simulink model "c28035solar_inverter"  (R2021b)
settings: Solver=FixedStepDiscrete  StartTime=0.0  StopTime=inf  FixedStep=1e-5  RelTol=1e-3  EnableMultiTasking=on
undefined symbols (not defined in the file or in its folder): Down, GPTRIP1SEL, GPTRIP2SEL, TZ1, TZ2, Up
libraries: c2802xlib x8, tiiqmathlib x6, simulink x5, c280xlib x3, c28xdmclib x2, c2000lib x1, demo_controls x1
settings Model: ExtModeTrigType=signal  ExtModeTrigDuration=10  ExtModeTrigDurationFloating=10  ExtModeTrigDelay=-2  ExtModeTrigDirection=either  ExtModeTrigLevel=0.500000  Creator=The MathWorks, Inc.  LastModifiedBy=The MathWorks, Inc.
settings SolverCC: AlgebraicLoopSolver=TrustRegion
settings DataIOCC: LimitDataPoints=on  SaveFormat=Array  SaveOutput=off  SaveTime=off  ReturnWorkspaceOutputs=off
settings OptimizationCC: DefaultParameterBehavior=Inlined  UseSpecifiedMinMax=on  StrengthReduction=on  PassReuseOutputArgsAs=Individual arguments  NoFixptDivByZeroProtection=on  EfficientFloat2IntCast=on  LifeSpan=1  MaxStackSize=512  EfficientTunableParamExpr=on
settings DebuggingCC: SolverPrmCheckMsg=warning  InheritedTsInSrcMsg=none  ParameterPrecisionLossMsg=none  AllowSymbolicDim=off  SFUnexpectedBacktrackingDiag=warning  SFNoUnconditionalDefaultTransitionDiag=warning  SFExecutionAtInitializationDiag=none  SFMachineParentedDataDiag=warning  ArithmeticOperatorsInVariantConditions=warning
settings HardwareCC: ProdBitPerChar=16  ProdBitPerInt=16  ProdBitPerPointer=16  ProdBitPerSizeT=32  ProdBitPerPtrDiffT=32  ProdLargestAtomicInteger=Integer  ProdLargestAtomicFloat=None  ProdWordSize=16  ProdHWDeviceType=Texas Instruments->C2000
settings ModelReferenceCC: PropagateSignalLabelsOutOfModel=off
settings SFSimCC: SimUseLocalCustomCode=off  MATLABDynamicMemAlloc=off  CustomCodeUndefinedFunction=UseInterfaceOnly
settings RTWCC: Description=Embedded Coder  SystemTargetFile=ert.tlc  HardwareBoard=TI Piccolo F2803x  TemplateMakefile=ert_default_tmf  RTWUseLocalCustomCode=off  Toolchain=Texas Instruments Code Composer Studio (C2000)  BuildConfiguration=Debug
settings CodeAppCC: IgnoreCustomStorageClasses=off  StateflowObjectComments=on
settings ERTTargetCC: CodeReplacementLibrary=TI C28x  UtilityFuncGeneration=Shared location  MultiwordLength=2048  CombineSignalStateStructs=on  SupportNonFinite=off  SupportComplex=off  SupportContinuousTime=on  ExtModeMexFile=TIC2000ExternalModeOpen  ExtModeMexArgs=1 65 115385 30  ExtModeIntrfLevel=Level2 - Open  ERTFilePackagingFormat=Compact  MemSecPackage=tic2000demospkg  MemSecFuncExecute=code_ramfuncs
settings ConfigComp: CovMetricSettings=dw  CovSaveCumulativeToWorkspaceVar=on  CovSaveSingleToWorkspaceVar=on  CovExternalEMLEnable=off  CovSFcnEnable=off
settings SimscapeCC: SimscapeNormalizeSystem=off
settings ConfigurationSet: Description=SimMechanics 2G

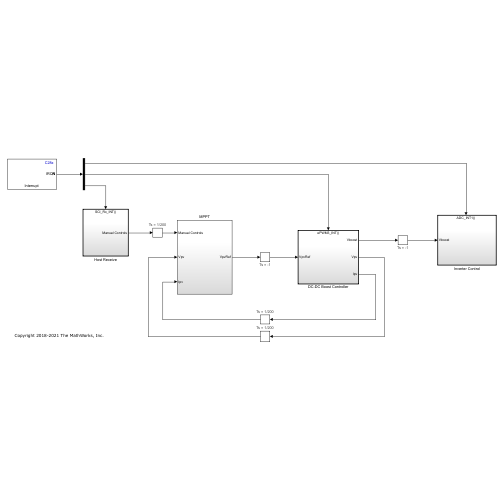
[thumbnail: Simulink's stored preview of the top-level diagram]
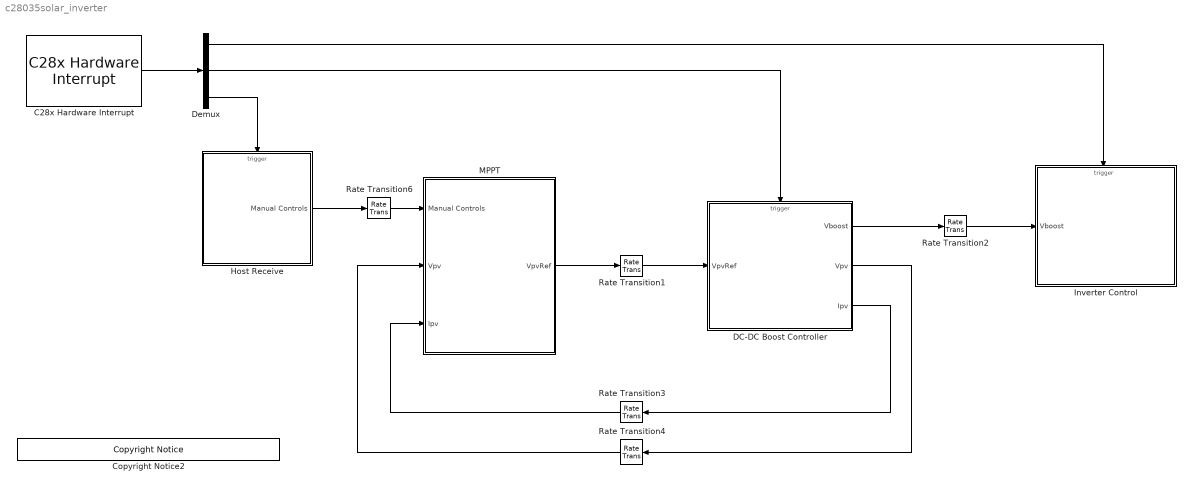
== system c28035solar_inverter ==
  C28x Hardware Interrupt : c2000lib/Scheduling/C28x Hardware Interrupt  irqnumbers=[1 3 9]  pienumbers=[1 3 1]  irqpriorities=[36 30 50]  irqpreempts=[1 0 0]  showinput=off  dspchiptype=C280X
      settings: SourceProductBaseCode=TIC2000
  Copyright Notice2 : demo_controls/Copyright Notice  year=2018  prod=tic2000
      settings: SourceProductBaseCode=ME
  DC-DC Boost Controller : Subsystem  TreatAsAtomicUnit=on
  Demux : Demux  Outputs=3
  Host Receive : Subsystem
  Inverter Control : Subsystem  TreatAsAtomicUnit=on
  MPPT : Subsystem
  Rate Transition1 : RateTransition  Deterministic=off
      settings: AttributesFormatString=Ts = %<OutPortSampleTime>
  Rate Transition2 : RateTransition  Deterministic=off
      settings: AttributesFormatString=Ts = %<OutPortSampleTime>
  Rate Transition3 : RateTransition  Deterministic=off  OutPortSampleTime=1/200
      settings: AttributesFormatString=Ts = %<OutPortSampleTime>
  Rate Transition4 : RateTransition  Deterministic=off  OutPortSampleTime=1/200
      settings: AttributesFormatString=Ts = %<OutPortSampleTime>
  Rate Transition6 : RateTransition  Deterministic=off  OutPortSampleTime=1/200
      settings: AttributesFormatString=Ts = %<OutPortSampleTime>
  wires:
  DC-DC Boost Controller/1(Vboost) -> Rate Transition2/1
  Demux/2 -> DC-DC Boost Controller/Trigger
  Rate Transition2/1 -> Inverter Control/1(Vboost)
  Demux/3 -> Host Receive/Trigger
  Rate Transition3/1 -> MPPT/3(Ipv)
  Rate Transition4/1 -> MPPT/2(Vpv)
  C28x Hardware Interrupt/1 -> Demux/1
  Host Receive/1(Manual Controls) -> Rate Transition6/1
  DC-DC Boost Controller/3(Ipv) -> Rate Transition3/1
  DC-DC Boost Controller/2(Vpv) -> Rate Transition4/1
  Rate Transition6/1 -> MPPT/1(Manual Controls)
  MPPT/1(VpvRef) -> Rate Transition1/1
  Demux/1 -> Inverter Control/Trigger
  Rate Transition1/1 -> DC-DC Boost Controller/1(VpvRef)

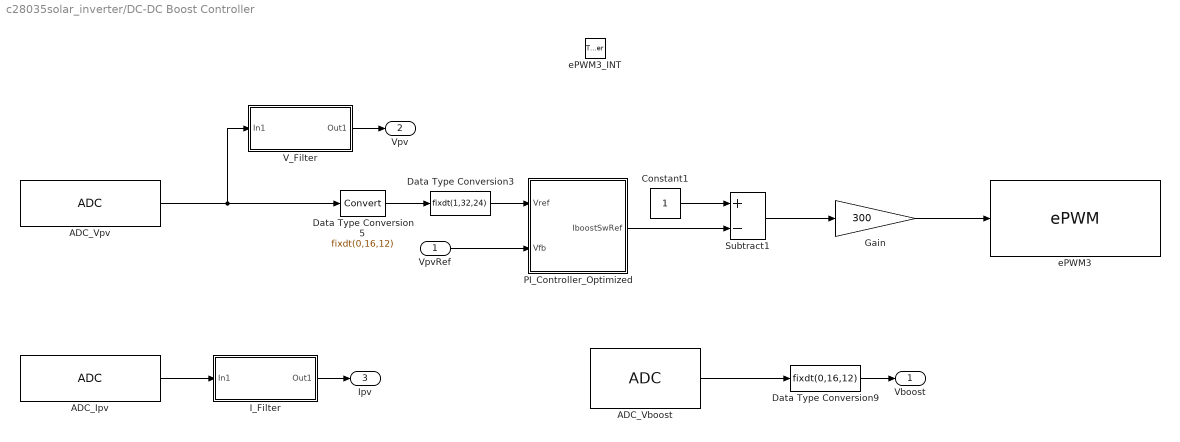
== system c28035solar_inverter/DC-DC Boost Controller ==
  VpvRef : Inport
  ePWM3_INT : TriggerPort  TriggerType=function-call  VariantControl=(inherit)
  ADC_Ipv : c2802xlib/ADC  blkParamProc=C2000  ADCModule=1  samplingMode=Single sample mode  ADCResolution=12-bit (Single-ended input)  useSOC1=SOC6  useSOC2=SOC0_SOC1  SOCAcquisitionWindow=7  SOCTriggerSource=ePWM3_ADCSOCA  SOCInterruptTrigger=No ADCINT  Ts=-1  dType=uint16  postInterrupt=off  interruptSel=ADCINT1  ADCINTContinuous=off  endma=off  chdma=1  conv1=ADCINA0  conv2=ADCINA0 and ADCINB0  conv1_Type4=ADCIN0  conv2_Type4=ADCIN0 and ADCIN1
  ADC_Vboost : c2802xlib/ADC  blkParamProc=C2000  ADCModule=1  samplingMode=Single sample mode  ADCResolution=12-bit (Single-ended input)  useSOC1=SOC5  useSOC2=SOC0_SOC1  SOCAcquisitionWindow=7  SOCTriggerSource=ePWM3_ADCSOCB  SOCInterruptTrigger=No ADCINT  Ts=-1  dType=uint16  postInterrupt=off  interruptSel=ADCINT1  ADCINTContinuous=off  endma=off  chdma=1  conv1=ADCINA2  conv2=ADCINA0 and ADCINB0  conv1_Type4=ADCIN0  conv2_Type4=ADCIN0 and ADCIN1
  ADC_Vpv : c2802xlib/ADC  blkParamProc=C2000  ADCModule=1  samplingMode=Single sample mode  ADCResolution=12-bit (Single-ended input)  useSOC1=SOC7  useSOC2=SOC0_SOC1  SOCAcquisitionWindow=7  SOCTriggerSource=ePWM3_ADCSOCA  SOCInterruptTrigger=No ADCINT  Ts=-1  dType=uint16  postInterrupt=off  interruptSel=ADCINT1  ADCINTContinuous=on  endma=off  chdma=1  conv1=ADCINA1  conv2=ADCINA0 and ADCINB0  conv1_Type4=ADCIN0  conv2_Type4=ADCIN0 and ADCIN1
  Constant1 : Constant  OutDataTypeStr=fixdt(1,32,24)  SampleTime=-1
  Data Type Conversion3 : DataTypeConversion  OutDataTypeStr=fixdt(1,32,24)
  Data Type Conversion5 : DataTypeConversion  OutDataTypeStr=fixdt(0,16,12)  ConvertRealWorld=Stored Integer (SI)  RndMeth=Simplest
      settings: AttributesFormatString=DataType = %<OutDataTypeStr>
  Data Type Conversion9 : DataTypeConversion  OutDataTypeStr=fixdt(0,16,12)  ConvertRealWorld=Stored Integer (SI)  RndMeth=Simplest
      settings: AttributesFormatString=DataType = %<OutDataTypeStr>
  Gain : Gain  Gain=300  ParamDataTypeStr=uint16  OutDataTypeStr=uint16  RndMeth=Simplest
  I_Filter : Subsystem
  PI_Controller_Optimized : Subsystem  VariantControl=Variant
  Subtract1 : Sum  Inputs=+-
  V_Filter : Subsystem
  ePWM3 : c2802xlib/ePWM  PwmType=C2000  useModule=ePWM3  ePWMxLINKTBPRD=Not Linked  periodUnits=Clock cycles  timerSource=Specify via dialog  timerPeriod_clk=300  timerPeriod_sec=0.0001  tbshadow=Counter equals to zero  countingMode=Up-Down  phaseActiveEnable=Set counter to phase value specified via dialog  phaseDirection=Count up after sync  phaseActive=4  synchronizationEnable=off  dcaevt1Sync=off  dcbevt1Sync=off  synchronizationOption=Disable  perSynchronizationOption=Counter equals to period (CTR=PRD)  clockPrescale=1  HSclockPrescale=1  enswap=off  ePWMxAStatus=on  ePWMxAactionLogic1=Do nothing  ePWMxAactionLogic2=Do nothing  ePWMxAactionLogic3=Set  ePWMxAactionLogic4=Clear  ePWMxAactionLogic5=Do nothing  ePWMxAactionLogic6=Do nothing  ePWMxACSFenable=off  ePWMxACSFvalue=Forcing disable  ePWMxASFreload=Zero  ePWMxBStatus=off  ePWMxBactionLogic1=Do nothing  ePWMxBactionLogic2=Do nothing  ePWMxBactionLogic3=Do nothing  ePWMxBactionLogic4=Do nothing  ePWMxBactionLogic5=Do nothing  ePWMxBactionLogic6=Do nothing  ePWMxBCSFenable=off  ePWMxBCSFvalue=Forcing disable  ePWMxBSFreload=Zero  ePWNxBOutWay=off  ePWMxLINKCMPA=Not Linked  CMPAUnits=Clock cycles  CMPASource=Input port  CMPAValue_per=0  CMPAValue_clk=300  enCMPAshadow=Counter equals to zero (CTR=Zero)  ePWMxLINKCMPB=Not Linked  CMPBUnits=Clock cycles  CMPBSource=Specify via dialog  CMPBValue_per=50  CMPBValue_clk=0  enCMPBshadow=Counter equals to zero (CTR=Zero)  ePWMxLINKCMPC=Not Linked  CMPCUnits=Clock cycles  CMPCSource=Specify via dialog  CMPCValue_per=50  CMPCValue_clk=32000  enCMPCshadow=Counter equals to zero (CTR=Zero)  ePWMxLINKCMPD=Not Linked  CMPDUnits=Clock cycles  CMPDSource=Specify via dialog  CMPDValue_per=50  CMPDValue_clk=32000  enCMPDshadow=Counter equals to zero (CTR=Zero)  enableDBePWMxA=on  enableDBePWMxB=on  enhalfcycle=off  DBpolarity=Active high (AH)  DBedgeDelay=Positive  DBSource_ePWMxA=ePWMxA  DBSource_ePWMxB=ePWMxA  DBPeriodUnits=Clock cycles  DBperiodSource=Specify via dialog  REDperiod=0  FEDperiod=30  REDperiod_sec=0  FEDperiod_sec=0  LoadModeDBRED=Immediate without using shadow  LoadModeDBFED=Immediate without using shadow  adcstartModuleA=on  adcrequestEventA=Second event  adcstartEventA=Counter is incrementing and equals to the compare B register (CTRU=CMPB)  adcstartEventA_type2=Digital Compare Module A Event 1 start of conversion (DCAEVT1.soc)  adcstartModuleB=on  adcrequestEventB=Second event  adcstartEventB=Counter equals to period (CTR=PRD)  adcstartEventB_type2=Counter equals to zero (CTR=Zero)  intEn=on  intPrd=Second event  intSel=Counter equals to period (CTR=PRD)  intSel_type2=Counter equals to zero (CTR=Zero)  hrpe=off  enHRPWM=off  HRPWM_LoadMode=Counter equals to period (CTR=PRD)  HRPWM_CTLMode=Duty or Period control mode  HRPWM_EDGMode=Falling edge  hrpeb=off  enHRPWMB=off  HRPWM_LoadModeB=Counter equals to zero (CTR=ZERO)  HRPWM_CTLModeB=Duty or Period control mode  HRPWM_EDGModeB=Both edge  enHRDBRED=off  enHRDBFED=off  enSFO=off  enautoconv=off  chopperEnable=off  chopperFrequency=1  chopperFirstwidth=1  chopperDuty=12.5%  tripZonesource=Specify via dialog  tzselOSHT1=off  tzselOSHT2=off  tzselOSHT3=off  tzselOSHDCAEV1=off  tzselOSHDCBEV1=off  tzselCBC1=off  tzselCBC2=off  tzselCBC3=off  tzselCBCDCAEV2=off  tzselCBCDCBEV2=off  tzselOSHT4=off  tzselOSHT5=off  tzselOSHT6=off  tzselCBC4=off  tzselCBC5=off  tzselCBC6=off  enTzOstIntr=off  enTzCbcIntr=off  enTzDCAEVT1Intr=off  enTzDCAEVT2Intr=off  enTzDCBEVT1Intr=off  enTzDCBEVT2Intr=off  ePWMxAforced=Low  ePWMxBforced=No action  DCAEVT1forced=No action  DCBEVT1forced=No action  DCAEVT2forced=No action  DCBEVT2forced=No action  dcah=COMP1OUT input  dcal=COMP1OUT input  dcbh=COMP2OUT input  dcbl=COMP3OUT input  dcah_type2=GPTRIP1SEL/(TZ1)  dcal_type2=GPTRIP2SEL/(TZ2)  dcbh_type2=GPTRIP1SEL/(TZ1)  dcbl_type2=GPTRIP2SEL/(TZ2)  gendcaevt1=DCAH=high and DCAL=don't care  gendcaevt2=Event disabled  gendcbevt1=Event disabled  gendcbevt2=Event disabled  dcaevt1src=DCAEVT1 with async  dcaevt2src=DCAEVT2 with sync  dcbevt1src=DCBEVT1 with sync  dcbevt2src=DCBEVT2 with sync  pulsesel=Counter equals to zero (CTR=Zero)  blankinv=off  blankoffset=0  blankwidth=0  evsrcsel=Filtered version of DCAEVT1 (DCAEVT1FILT)  encape=off
  Vboost : Outport  VectorParamsAs1DForOutWhenUnconnected=off
  Vpv : Outport  Port=2  VectorParamsAs1DForOutWhenUnconnected=off
  Ipv : Outport  Port=3  VectorParamsAs1DForOutWhenUnconnected=off
  wires:
  Gain/1 -> ePWM3/1
  ADC_Vboost/1 -> Data Type Conversion9/1
  Data Type Conversion5/1 -> Data Type Conversion3/1
  Data Type Conversion3/1 -> PI_Controller_Optimized/1(Vref)
  ADC_Ipv/1 -> I_Filter/1(In1)
  ADC_Vpv/1 -> V_Filter/1(In1), Data Type Conversion5/1
  I_Filter/1(Out1) -> Ipv/1
  Data Type Conversion9/1 -> Vboost/1
  VpvRef/1 -> PI_Controller_Optimized/2(Vfb)
  V_Filter/1(Out1) -> Vpv/1
  Constant1/1 -> Subtract1/1
  PI_Controller_Optimized/1(IboostSwRef) -> Subtract1/2
  Subtract1/1 -> Gain/1

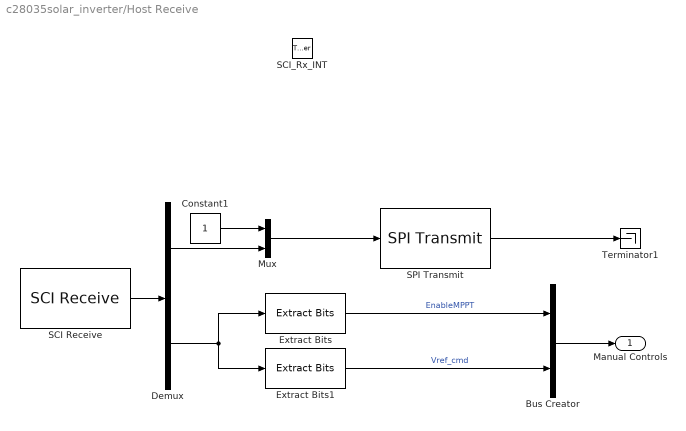
== system c28035solar_inverter/Host Receive ==
  SCI_Rx_INT : TriggerPort  TriggerType=function-call  VariantControl=Variant  PortDimensions=1
  Bus Creator : BusCreator  Inputs=2
  Constant1 : Constant  OutDataTypeStr=uint16  SampleTime=-1
  Demux : Demux  Outputs=2
  Extract Bits : simulink/Logic and Bit Operations/Extract Bits  bitsToExtract=Upper half  numBits=8  bitIdxRange=[0 7]  outScalingMode=Treat bit field as an integer
  Extract Bits1 : simulink/Logic and Bit Operations/Extract Bits  bitsToExtract=Lower half  numBits=8  bitIdxRange=[0 7]  outScalingMode=Treat bit field as an integer
  Mux : Mux  Inputs=2
  SCI Receive : c280xlib/SCI Receive  sciModule=A  dataHead=''  dataTail=''  dataType=uint16  dataDim=2  initValue=0  errOption=Output the last received value  errValue=0  sampleTime=-1  outputStatus=off  postInterrupt=on  numFifo=4
      settings: SourceProductBaseCode=TIC2000
  SPI Transmit : c280xlib/SPI Transmit  SPISelect=SPI_B  ClockPolarity=Rising_edge  ClockPhase=No_delay  SPIModule=uint32(0)  Mode=Master  BusSpeed=uint32(1000000)  FirstBitToTransfer=Most significant bit (MSB)  ClockMode=0  BlockFunction=Write  EnableRegisterAddress=on  RegisterAddress=0  OutputDataType=int8  OutputDataLength=1  BlockingMode=off  DataBits=16  UseCustomSSPin=Provided by the SPI peripheral  ActiveLowSSPin=Active low  Pin=0
      settings: SourceProductBaseCode=TIC2000
  Terminator1 : Terminator
  Manual Controls : Outport  VectorParamsAs1DForOutWhenUnconnected=off
  wires:
  Constant1/1 -> Mux/1
  Mux/1 -> SPI Transmit/1
  SPI Transmit/1 -> Terminator1/1
  Demux/2 -> Extract Bits/1, Extract Bits1/1
  Extract Bits/1 -> Bus Creator/1  "EnableMPPT"
  Extract Bits1/1 -> Bus Creator/2  "Vref_cmd"
  Bus Creator/1 -> Manual Controls/1
  SCI Receive/1 -> Demux/1
  Demux/1 -> Mux/2

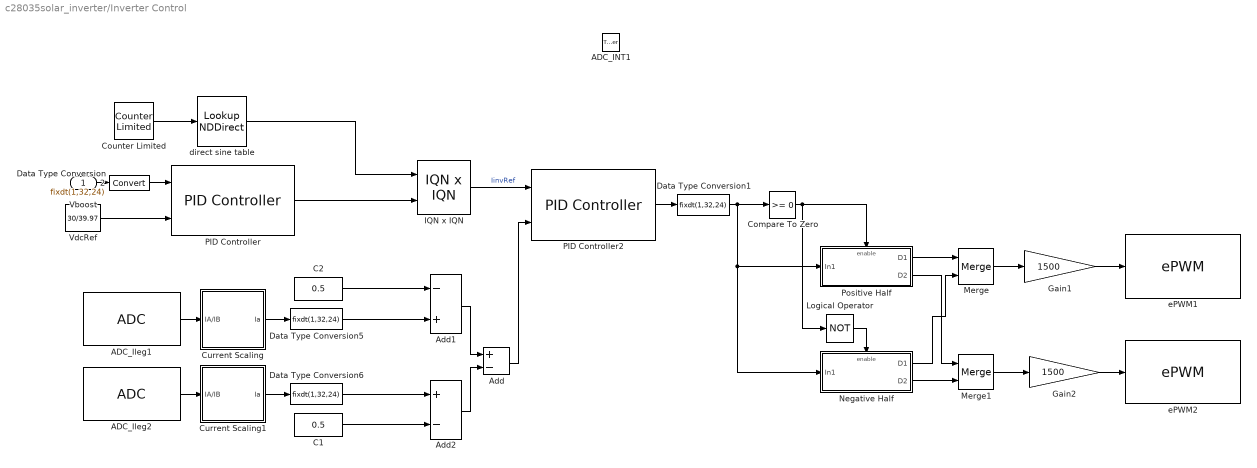
== system c28035solar_inverter/Inverter Control ==
  Vboost : Inport
  ADC_INT1 : TriggerPort  TriggerType=function-call  VariantControl=(inherit)
  ADC_Ileg1 : c2802xlib/ADC  blkParamProc=C2000  ADCModule=1  samplingMode=Single sample mode  ADCResolution=12-bit (Single-ended input)  useSOC1=SOC3  useSOC2=SOC0_SOC1  SOCAcquisitionWindow=7  SOCTriggerSource=ePWM1_ADCSOCA  SOCInterruptTrigger=No ADCINT  Ts=-1  dType=uint16  postInterrupt=on  interruptSel=ADCINT1  ADCINTContinuous=on  endma=off  chdma=1  conv1=ADCINA4  conv2=ADCINA0 and ADCINB0  conv1_Type4=ADCIN0  conv2_Type4=ADCIN0 and ADCIN1
  ADC_Ileg2 : c2802xlib/ADC  blkParamProc=C2000  ADCModule=1  samplingMode=Single sample mode  ADCResolution=12-bit (Single-ended input)  useSOC1=SOC4  useSOC2=SOC0_SOC1  SOCAcquisitionWindow=7  SOCTriggerSource=ePWM1_ADCSOCA  SOCInterruptTrigger=No ADCINT  Ts=-1  dType=uint16  postInterrupt=off  interruptSel=ADCINT1  ADCINTContinuous=off  endma=off  chdma=1  conv1=ADCINA6  conv2=ADCINA0 and ADCINB0  conv1_Type4=ADCIN0  conv2_Type4=ADCIN0 and ADCIN1
  Add : Sum  Inputs=+-
  Add1 : Sum  Inputs=-+
  Add2 : Sum  Inputs=+-
  C1 : Constant  Value=0.5  OutDataTypeStr=fixdt(1,32,24)  SampleTime=-1
  C2 : Constant  Value=0.5  OutDataTypeStr=fixdt(1,32,24)  SampleTime=-1
  Compare To Zero : simulink/Logic and Bit Operations/Compare To Zero  relop=>=  OutDataTypeStr=boolean
  Counter Limited : simulink/Sources/Counter Limited  uplimit=400  tsamp=-1
  Current Scaling : Subsystem
  Current Scaling1 : Subsystem
  Data Type Conversion1 : DataTypeConversion  OutDataTypeStr=fixdt(1,32,24)
  Data Type Conversion2 : DataTypeConversion  OutDataTypeStr=fixdt(1,32,24)
  Data Type Conversion5 : DataTypeConversion  OutDataTypeStr=fixdt(1,32,24)  ConvertRealWorld=Stored Integer (SI)
  Data Type Conversion6 : DataTypeConversion  OutDataTypeStr=fixdt(1,32,24)  ConvertRealWorld=Stored Integer (SI)
  Gain1 : Gain  Gain=1500  ParamDataTypeStr=uint16  OutDataTypeStr=uint16  RndMeth=Simplest
  Gain2 : Gain  Gain=1500  ParamDataTypeStr=uint16  OutDataTypeStr=uint16  RndMeth=Simplest
  IQN x IQN : tiiqmathlib/IQN x IQN  multiplyOption=Multiply
      settings: SourceProductBaseCode=TIC2000
  Logical Operator : Logic  Operator=NOT  AllPortsSameDT=off  OutDataTypeStr=boolean
  Merge : Merge
  Merge1 : Merge
  Negative Half : Subsystem  TreatAsAtomicUnit=on
  PID Controller : c28xdmclib/PID Controller  proportionalGain=3  integralGain=0.005  correctionGain=1  derivativeGain=0  minOutput=0  maxOutput=0.95
      settings: SourceProductBaseCode=TIC2000
  PID Controller2 : c28xdmclib/PID Controller  proportionalGain=0.25  integralGain=0.2  correctionGain=1  derivativeGain=0  minOutput=-1  maxOutput=1
      settings: SourceProductBaseCode=TIC2000
  Positive Half : Subsystem  TreatAsAtomicUnit=on
  VdcRef : Constant  Value=30/39.97  OutDataTypeStr=fixdt(1,32,24)  SampleTime=-1
  direct sine table : LookupNDDirect  NumberOfTableDimensions=1  Table=sin( 2*pi * (0:400)/400+90/180)'  TableDataTypeStr=fixdt(1,32,24)
  ePWM1 : c2802xlib/ePWM  PwmType=C2000  useModule=ePWM1  ePWMxLINKTBPRD=Not Linked  periodUnits=Clock cycles  timerSource=Specify via dialog  timerPeriod_clk=1500  timerPeriod_sec=0.0001  tbshadow=Counter equals to zero  countingMode=Up-Down  phaseActiveEnable=Disable  phaseDirection=Count down after sync  phaseActive=750  synchronizationEnable=off  dcaevt1Sync=off  dcbevt1Sync=off  synchronizationOption=Counter equals to zero (CTR=Zero)  perSynchronizationOption=Counter equals to period (CTR=PRD)  clockPrescale=1  HSclockPrescale=1  enswap=off  ePWMxAStatus=on  ePWMxAactionLogic1=Do nothing  ePWMxAactionLogic2=Do nothing  ePWMxAactionLogic3=Clear  ePWMxAactionLogic4=Set  ePWMxAactionLogic5=Do nothing  ePWMxAactionLogic6=Do nothing  ePWMxACSFenable=off  ePWMxACSFvalue=Forcing disable  ePWMxASFreload=Zero  ePWMxBStatus=off  ePWMxBactionLogic1=Do nothing  ePWMxBactionLogic2=Do nothing  ePWMxBactionLogic3=Do nothing  ePWMxBactionLogic4=Do nothing  ePWMxBactionLogic5=Do nothing  ePWMxBactionLogic6=Do nothing  ePWMxBCSFenable=off  ePWMxBCSFvalue=Forcing disable  ePWMxBSFreload=Zero  ePWNxBOutWay=on  ePWMxLINKCMPA=Not Linked  CMPAUnits=Clock cycles  CMPASource=Input port  CMPAValue_per=0  CMPAValue_clk=750  enCMPAshadow=Counter equals to zero (CTR=Zero)  ePWMxLINKCMPB=Not Linked  CMPBUnits=Clock cycles  CMPBSource=Specify via dialog  CMPBValue_per=50  CMPBValue_clk=0  enCMPBshadow=Counter equals to zero (CTR=Zero)  ePWMxLINKCMPC=Not Linked  CMPCUnits=Clock cycles  CMPCSource=Specify via dialog  CMPCValue_per=50  CMPCValue_clk=32000  enCMPCshadow=Counter equals to zero (CTR=Zero)  ePWMxLINKCMPD=Not Linked  CMPDUnits=Clock cycles  CMPDSource=Specify via dialog  CMPDValue_per=50  CMPDValue_clk=32000  enCMPDshadow=Counter equals to zero (CTR=Zero)  enableDBePWMxA=on  enableDBePWMxB=on  enhalfcycle=off  DBpolarity=Active high complementary (AHC)  DBedgeDelay=Positive  DBSource_ePWMxA=ePWMxA  DBSource_ePWMxB=ePWMxB  DBPeriodUnits=Clock cycles  DBperiodSource=Specify via dialog  REDperiod=20  FEDperiod=20  REDperiod_sec=0  FEDperiod_sec=0  LoadModeDBRED=Immediate without using shadow  LoadModeDBFED=Immediate without using shadow  adcstartModuleA=on  adcrequestEventA=First event  adcstartEventA=Counter equals to zero (CTR=Zero)  adcstartEventA_type2=Digital Compare Module A Event 1 start of conversion (DCAEVT1.soc)  adcstartModuleB=off  adcrequestEventB=First event  adcstartEventB=Counter equals to zero (CTR=Zero)  adcstartEventB_type2=Counter equals to zero (CTR=Zero)  intEn=off  intPrd=First event  intSel=Counter equals to period (CTR=PRD)  intSel_type2=Counter equals to zero (CTR=Zero)  hrpe=off  enHRPWM=off  HRPWM_LoadMode=Counter equals to period (CTR=PRD)  HRPWM_CTLMode=Duty or Period control mode  HRPWM_EDGMode=Falling edge  hrpeb=off  enHRPWMB=off  HRPWM_LoadModeB=Counter equals to zero (CTR=ZERO)  HRPWM_CTLModeB=Duty or Period control mode  HRPWM_EDGModeB=Both edge  enHRDBRED=off  enHRDBFED=off  enSFO=off  enautoconv=off  chopperEnable=off  chopperFrequency=1  chopperFirstwidth=1  chopperDuty=12.5%  tripZonesource=Specify via dialog  tzselOSHT1=off  tzselOSHT2=off  tzselOSHT3=off  tzselOSHDCAEV1=off  tzselOSHDCBEV1=off  tzselCBC1=off  tzselCBC2=off  tzselCBC3=off  tzselCBCDCAEV2=off  tzselCBCDCBEV2=off  tzselOSHT4=off  tzselOSHT5=off  tzselOSHT6=off  tzselCBC4=off  tzselCBC5=off  tzselCBC6=off  enTzOstIntr=off  enTzCbcIntr=off  enTzDCAEVT1Intr=off  enTzDCAEVT2Intr=off  enTzDCBEVT1Intr=off  enTzDCBEVT2Intr=off  ePWMxAforced=Low  ePWMxBforced=No action  DCAEVT1forced=No action  DCBEVT1forced=No action  DCAEVT2forced=No action  DCBEVT2forced=No action  dcah=COMP1OUT input  dcal=COMP3OUT input  dcbh=COMP3OUT input  dcbl=COMP2OUT input  dcah_type2=GPTRIP1SEL/(TZ1)  dcal_type2=GPTRIP2SEL/(TZ2)  dcbh_type2=GPTRIP1SEL/(TZ1)  dcbl_type2=GPTRIP2SEL/(TZ2)  gendcaevt1=DCAH=high and DCAL=don't care  gendcaevt2=Event disabled  gendcbevt1=Event disabled  gendcbevt2=Event disabled  dcaevt1src=DCAEVT1 with async  dcaevt2src=DCAEVT2 with sync  dcbevt1src=DCBEVT1 with sync  dcbevt2src=DCBEVT2 with sync  pulsesel=Counter equals to zero (CTR=Zero)  blankinv=off  blankoffset=0  blankwidth=0  evsrcsel=Filtered version of DCAEVT1 (DCAEVT1FILT)  encape=off
  ePWM2 : c2802xlib/ePWM  PwmType=C2000  useModule=ePWM2  ePWMxLINKTBPRD=Not Linked  periodUnits=Clock cycles  timerSource=Specify via dialog  timerPeriod_clk=1500  timerPeriod_sec=0.0001  tbshadow=Counter equals to zero  countingMode=Up-Down  phaseActiveEnable=Set counter to phase value specified via dialog  phaseDirection=Count up after sync  phaseActive=2  synchronizationEnable=off  dcaevt1Sync=off  dcbevt1Sync=off  synchronizationOption=Counter equals to zero (CTR=Zero)  perSynchronizationOption=Counter equals to period (CTR=PRD)  clockPrescale=1  HSclockPrescale=1  enswap=off  ePWMxAStatus=on  ePWMxAactionLogic1=Do nothing  ePWMxAactionLogic2=Do nothing  ePWMxAactionLogic3=Clear  ePWMxAactionLogic4=Set  ePWMxAactionLogic5=Do nothing  ePWMxAactionLogic6=Do nothing  ePWMxACSFenable=off  ePWMxACSFvalue=Forcing disable  ePWMxASFreload=Zero  ePWMxBStatus=off  ePWMxBactionLogic1=Do nothing  ePWMxBactionLogic2=Do nothing  ePWMxBactionLogic3=Do nothing  ePWMxBactionLogic4=Do nothing  ePWMxBactionLogic5=Do nothing  ePWMxBactionLogic6=Do nothing  ePWMxBCSFenable=off  ePWMxBCSFvalue=Forcing disable  ePWMxBSFreload=Zero  ePWNxBOutWay=on  ePWMxLINKCMPA=Not Linked  CMPAUnits=Clock cycles  CMPASource=Input port  CMPAValue_per=0  CMPAValue_clk=750  enCMPAshadow=Counter equals to period (CTR=PRD)  ePWMxLINKCMPB=Not Linked  CMPBUnits=Clock cycles  CMPBSource=Specify via dialog  CMPBValue_per=50  CMPBValue_clk=0  enCMPBshadow=Counter equals to zero (CTR=Zero)  ePWMxLINKCMPC=Not Linked  CMPCUnits=Clock cycles  CMPCSource=Specify via dialog  CMPCValue_per=50  CMPCValue_clk=32000  enCMPCshadow=Counter equals to zero (CTR=Zero)  ePWMxLINKCMPD=Not Linked  CMPDUnits=Clock cycles  CMPDSource=Specify via dialog  CMPDValue_per=50  CMPDValue_clk=32000  enCMPDshadow=Counter equals to zero (CTR=Zero)  enableDBePWMxA=on  enableDBePWMxB=on  enhalfcycle=off  DBpolarity=Active high complementary (AHC)  DBedgeDelay=Positive  DBSource_ePWMxA=ePWMxA  DBSource_ePWMxB=ePWMxB  DBPeriodUnits=Clock cycles  DBperiodSource=Specify via dialog  REDperiod=20  FEDperiod=20  REDperiod_sec=0  FEDperiod_sec=0  LoadModeDBRED=Immediate without using shadow  LoadModeDBFED=Immediate without using shadow  adcstartModuleA=on  adcrequestEventA=First event  adcstartEventA=Counter equals to zero (CTR=Zero)  adcstartEventA_type2=Digital Compare Module A Event 1 start of conversion (DCAEVT1.soc)  adcstartModuleB=off  adcrequestEventB=First event  adcstartEventB=Counter equals to zero (CTR=Zero)  adcstartEventB_type2=Counter equals to zero (CTR=Zero)  intEn=off  intPrd=First event  intSel=Counter equals to period (CTR=PRD)  intSel_type2=Counter equals to zero (CTR=Zero)  hrpe=off  enHRPWM=off  HRPWM_LoadMode=Counter equals to period (CTR=PRD)  HRPWM_CTLMode=Duty or Period control mode  HRPWM_EDGMode=Falling edge  hrpeb=off  enHRPWMB=off  HRPWM_LoadModeB=Counter equals to zero (CTR=ZERO)  HRPWM_CTLModeB=Duty or Period control mode  HRPWM_EDGModeB=Both edge  enHRDBRED=off  enHRDBFED=off  enSFO=off  enautoconv=off  chopperEnable=off  chopperFrequency=1  chopperFirstwidth=1  chopperDuty=12.5%  tripZonesource=Specify via dialog  tzselOSHT1=off  tzselOSHT2=off  tzselOSHT3=off  tzselOSHDCAEV1=off  tzselOSHDCBEV1=off  tzselCBC1=off  tzselCBC2=off  tzselCBC3=off  tzselCBCDCAEV2=off  tzselCBCDCBEV2=off  tzselOSHT4=off  tzselOSHT5=off  tzselOSHT6=off  tzselCBC4=off  tzselCBC5=off  tzselCBC6=off  enTzOstIntr=off  enTzCbcIntr=off  enTzDCAEVT1Intr=off  enTzDCAEVT2Intr=off  enTzDCBEVT1Intr=off  enTzDCBEVT2Intr=off  ePWMxAforced=Low  ePWMxBforced=No action  DCAEVT1forced=No action  DCBEVT1forced=No action  DCAEVT2forced=No action  DCBEVT2forced=No action  dcah=COMP1OUT input  dcal=COMP2OUT input  dcbh=COMP1OUT input  dcbl=COMP3OUT input  dcah_type2=GPTRIP1SEL/(TZ1)  dcal_type2=GPTRIP2SEL/(TZ2)  dcbh_type2=GPTRIP1SEL/(TZ1)  dcbl_type2=GPTRIP2SEL/(TZ2)  gendcaevt1=DCAH=high and DCAL=don't care  gendcaevt2=Event disabled  gendcbevt1=Event disabled  gendcbevt2=Event disabled  dcaevt1src=DCAEVT1 with async  dcaevt2src=DCAEVT2 with sync  dcbevt1src=DCBEVT1 with sync  dcbevt2src=DCBEVT2 with sync  pulsesel=Counter equals to zero (CTR=Zero)  blankinv=off  blankoffset=0  blankwidth=0  evsrcsel=Filtered version of DCAEVT1 (DCAEVT1FILT)  encape=off
  wires:
  Gain1/1 -> ePWM1/1
  Gain2/1 -> ePWM2/1
  ADC_Ileg1/1 -> Current Scaling/1(IA/IB)
  ADC_Ileg2/1 -> Current Scaling1/1(IA/IB)
  Current Scaling/1(Ia) -> Data Type Conversion5/1
  Current Scaling1/1(Ia) -> Data Type Conversion6/1
  Data Type Conversion5/1 -> Add1/2
  C2/1 -> Add1/1
  Add1/1 -> Add/1
  Data Type Conversion6/1 -> Add2/1
  Add2/1 -> Add/2
  PID Controller/1 -> IQN x IQN/2
  direct sine table/1 -> IQN x IQN/1
  Counter Limited/1 -> direct sine table/1
  Add/1 -> PID Controller2/2
  PID Controller2/1 -> Data Type Conversion1/1
  IQN x IQN/1 -> PID Controller2/1  "IinvRef"
  C1/1 -> Add2/2
  Logical Operator/1 -> Negative Half/Enable
  Compare To Zero/1 -> Positive Half/Enable, Logical Operator/1
  Positive Half/1(D1) -> Merge/1
  Data Type Conversion1/1 -> Compare To Zero/1, Negative Half/1(In1), Positive Half/1(In1)
  Negative Half/2(D2) -> Merge1/2
  Merge/1 -> Gain1/1
  Merge1/1 -> Gain2/1
  VdcRef/1 -> PID Controller/2
  Data Type Conversion2/1 -> PID Controller/1
  Vboost/1 -> Data Type Conversion2/1
  Positive Half/2(D2) -> Merge1/1
  Negative Half/1(D1) -> Merge/2

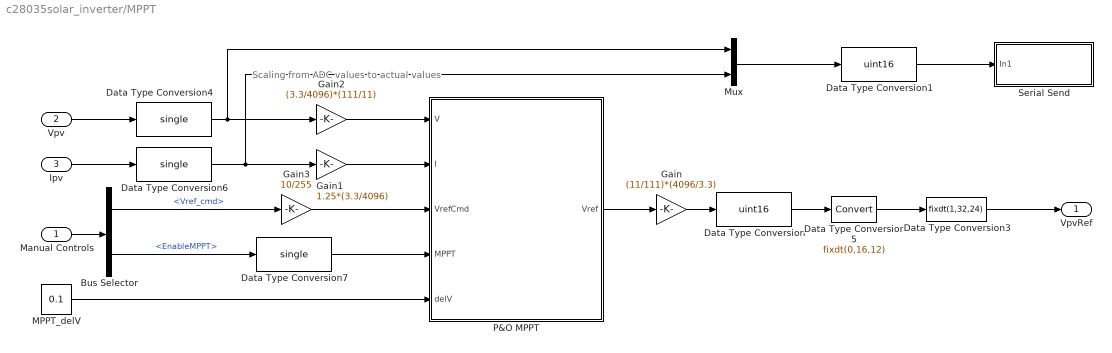
== system c28035solar_inverter/MPPT ==
  note: Scaling from ADC values to actual values
  Manual Controls : Inport
  Vpv : Inport  Port=2
  Ipv : Inport  Port=3
  Bus Selector : BusSelector  OutputSignals=Vref_cmd,EnableMPPT
  Data Type Conversion : DataTypeConversion  OutDataTypeStr=uint16  RndMeth=Nearest
  Data Type Conversion1 : DataTypeConversion  OutDataTypeStr=uint16  RndMeth=Convergent
  Data Type Conversion3 : DataTypeConversion  OutDataTypeStr=fixdt(1,32,24)
  Data Type Conversion4 : DataTypeConversion  OutDataTypeStr=single
  Data Type Conversion5 : DataTypeConversion  OutDataTypeStr=fixdt(0,16,12)  ConvertRealWorld=Stored Integer (SI)  RndMeth=Simplest
      settings: AttributesFormatString=DataType = %<OutDataTypeStr>
  Data Type Conversion6 : DataTypeConversion  OutDataTypeStr=single
  Data Type Conversion7 : DataTypeConversion  OutDataTypeStr=single
  Gain : Gain  Gain=(11/111)*(4096/3.3)
  Gain1 : Gain  Gain=1.25*(3.3/4096)
  Gain2 : Gain  Gain=(3.3/4096)*(111/11)  OutDataTypeStr=single
  Gain3 : Gain  Gain=10/255  OutDataTypeStr=single
  MPPT_delV : Constant  Value=0.1  OutDataTypeStr=single  SampleTime=-1
  Mux : Mux  Inputs=2
  P&O MPPT : Stateflow chart  TreatAsAtomicUnit=on
  Serial Send : Subsystem
  VpvRef : Outport  VectorParamsAs1DForOutWhenUnconnected=off
  wires:
  P&O MPPT/1(Vref) -> Gain/1
  Vpv/1 -> Data Type Conversion4/1
  Gain1/1 -> P&O MPPT/2(I)
  Data Type Conversion/1 -> Data Type Conversion5/1
  Data Type Conversion5/1 -> Data Type Conversion3/1
  Data Type Conversion4/1 -> Mux/1, Gain2/1
  Ipv/1 -> Data Type Conversion6/1
  Data Type Conversion6/1 -> Mux/2, Gain1/1
  Gain2/1 -> P&O MPPT/1(V)
  Data Type Conversion3/1 -> VpvRef/1
  Data Type Conversion1/1 -> Serial Send/1(In1)
  Mux/1 -> Data Type Conversion1/1
  Manual Controls/1 -> Bus Selector/1
  Bus Selector/2 -> Data Type Conversion7/1  "<EnableMPPT>"
  Bus Selector/1 -> Gain3/1  "<Vref_cmd>"
  Gain3/1 -> P&O MPPT/3(VrefCmd)
  Data Type Conversion7/1 -> P&O MPPT/4(MPPT)
  Gain/1 -> Data Type Conversion/1
  MPPT_delV/1 -> P&O MPPT/5(delV)

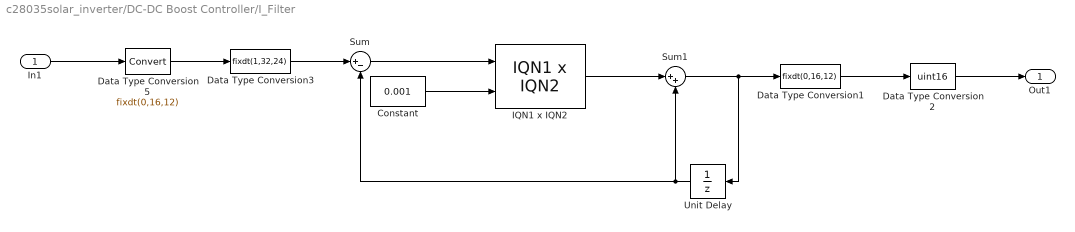
== system c28035solar_inverter/DC-DC Boost Controller/I_Filter ==
  In1 : Inport  OutDataTypeStr=uint16
  Constant : Constant  Value=0.001  OutDataTypeStr=fixdt(1,32,30)  SampleTime=-1
  Data Type Conversion1 : DataTypeConversion  OutDataTypeStr=fixdt(0,16,12)
  Data Type Conversion2 : DataTypeConversion  OutDataTypeStr=uint16  ConvertRealWorld=Stored Integer (SI)  RndMeth=Simplest
      settings: AttributesFormatString=DataType = %<OutDataTypeStr>
  Data Type Conversion3 : DataTypeConversion  OutDataTypeStr=fixdt(1,32,24)
  Data Type Conversion5 : DataTypeConversion  OutDataTypeStr=fixdt(0,16,12)  ConvertRealWorld=Stored Integer (SI)  RndMeth=Simplest
      settings: AttributesFormatString=DataType = %<OutDataTypeStr>
  IQN1 x IQN2 : tiiqmathlib/IQN1 x IQN2  Q=24
      settings: SourceProductBaseCode=TIC2000
  Sum : Sum  Inputs=|+-
  Sum1 : Sum  Inputs=|++
  Unit Delay : UnitDelay  SampleTime=-1  HasFrameUpgradeWarning=on
  Out1 : Outport  OutDataTypeStr=uint16  VectorParamsAs1DForOutWhenUnconnected=off
  wires:
  Data Type Conversion2/1 -> Out1/1
  Data Type Conversion1/1 -> Data Type Conversion2/1
  Data Type Conversion3/1 -> Sum/1
  In1/1 -> Data Type Conversion5/1
  Data Type Conversion5/1 -> Data Type Conversion3/1
  Constant/1 -> IQN1 x IQN2/2
  Unit Delay/1 -> Sum1/2, Sum/2
  Sum1/1 -> Data Type Conversion1/1, Unit Delay/1
  IQN1 x IQN2/1 -> Sum1/1
  Sum/1 -> IQN1 x IQN2/1

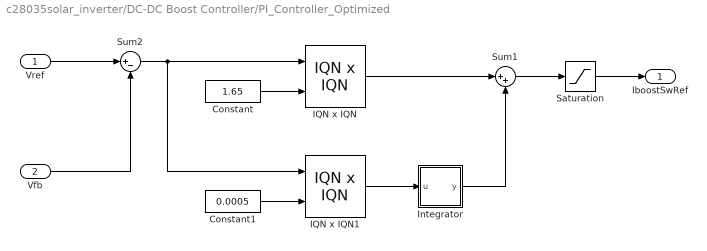
== system c28035solar_inverter/DC-DC Boost Controller/PI_Controller_Optimized ==
  Vref : Inport
  Vfb : Inport  Port=2
  Constant : Constant  Value=1.65  OutDataTypeStr=fixdt(1,32,24)  SampleTime=-1
      settings: AttributesFormatString=DataType = %<OutDataTypeStr>
  Constant1 : Constant  Value=0.0005  OutDataTypeStr=fixdt(1,32,24)  SampleTime=-1
      settings: AttributesFormatString=DataType = %<OutDataTypeStr>
  IQN x IQN : tiiqmathlib/IQN x IQN  multiplyOption=Multiply
      settings: SourceProductBaseCode=TIC2000
  IQN x IQN1 : tiiqmathlib/IQN x IQN  multiplyOption=Multiply
      settings: SourceProductBaseCode=TIC2000
  Integrator : Subsystem
  Saturation : Saturate  UpperLimit=1  LowerLimit=0.1  RndMeth=Simplest
      settings: AttributesFormatString=|
      | ULim = %<UpperLimit>
      | LLim = %<LowerLimit>
  Sum1 : Sum  Inputs=|++  RndMeth=Simplest  SaturateOnIntegerOverflow=on  OutDataTypeStr=Inherit: Same as first input
  Sum2 : Sum  Inputs=|+-  RndMeth=Simplest  OutDataTypeStr=Inherit: Same as first input
  IboostSwRef : Outport  VectorParamsAs1DForOutWhenUnconnected=off
  wires:
  Vref/1 -> Sum2/1
  Saturation/1 -> IboostSwRef/1
  Vfb/1 -> Sum2/2
  IQN x IQN/1 -> Sum1/1
  Sum1/1 -> Saturation/1
  Constant/1 -> IQN x IQN/2
  IQN x IQN1/1 -> Integrator/1(u)
  Constant1/1 -> IQN x IQN1/2
  Sum2/1 -> IQN x IQN1/1, IQN x IQN/1
  Integrator/1(y) -> Sum1/2

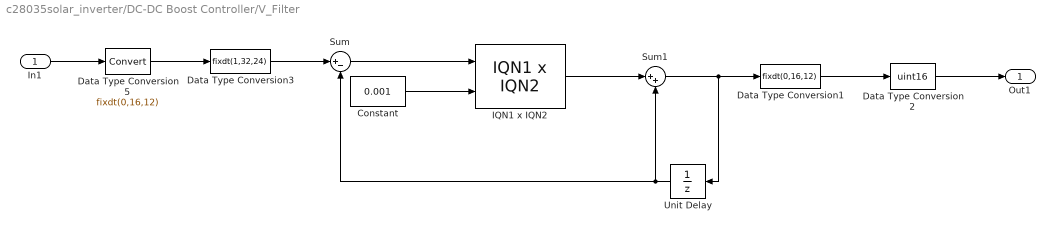
== system c28035solar_inverter/DC-DC Boost Controller/V_Filter ==
  In1 : Inport  OutDataTypeStr=uint16
  Constant : Constant  Value=0.001  OutDataTypeStr=fixdt(1,32,30)  SampleTime=-1
  Data Type Conversion1 : DataTypeConversion  OutDataTypeStr=fixdt(0,16,12)
  Data Type Conversion2 : DataTypeConversion  OutDataTypeStr=uint16  ConvertRealWorld=Stored Integer (SI)  RndMeth=Simplest
      settings: AttributesFormatString=DataType = %<OutDataTypeStr>
  Data Type Conversion3 : DataTypeConversion  OutDataTypeStr=fixdt(1,32,24)
  Data Type Conversion5 : DataTypeConversion  OutDataTypeStr=fixdt(0,16,12)  ConvertRealWorld=Stored Integer (SI)  RndMeth=Simplest
      settings: AttributesFormatString=DataType = %<OutDataTypeStr>
  IQN1 x IQN2 : tiiqmathlib/IQN1 x IQN2  Q=24
      settings: SourceProductBaseCode=TIC2000
  Sum : Sum  Inputs=|+-  OutDataTypeStr=fixdt(1,32,24)
  Sum1 : Sum  Inputs=|++
  Unit Delay : UnitDelay  SampleTime=-1  HasFrameUpgradeWarning=on
  Out1 : Outport  OutDataTypeStr=uint16  VectorParamsAs1DForOutWhenUnconnected=off
  wires:
  Sum/1 -> IQN1 x IQN2/1
  IQN1 x IQN2/1 -> Sum1/1
  Sum1/1 -> Unit Delay/1, Data Type Conversion1/1
  Unit Delay/1 -> Sum/2, Sum1/2
  Constant/1 -> IQN1 x IQN2/2
  Data Type Conversion5/1 -> Data Type Conversion3/1
  In1/1 -> Data Type Conversion5/1
  Data Type Conversion3/1 -> Sum/1
  Data Type Conversion1/1 -> Data Type Conversion2/1
  Data Type Conversion2/1 -> Out1/1

== system c28035solar_inverter/Inverter Control/Current Scaling ==
  IA/IB : Inport
  Data Type Conversion : DataTypeConversion  OutDataTypeStr=int32  ConvertRealWorld=Stored Integer (SI)
  Shift Arithmetic : ArithShift  BitShiftNumber=-12
  Ia : Outport  VectorParamsAs1DForOutWhenUnconnected=off
  wires:
  IA/IB/1 -> Data Type Conversion/1
  Shift Arithmetic/1 -> Ia/1
  Data Type Conversion/1 -> Shift Arithmetic/1

== system c28035solar_inverter/Inverter Control/Current Scaling1 ==
  IA/IB : Inport
  Data Type Conversion : DataTypeConversion  OutDataTypeStr=int32  ConvertRealWorld=Stored Integer (SI)
  Shift Arithmetic : ArithShift  BitShiftNumber=-12
  Ia : Outport  VectorParamsAs1DForOutWhenUnconnected=off
  wires:
  IA/IB/1 -> Data Type Conversion/1
  Shift Arithmetic/1 -> Ia/1
  Data Type Conversion/1 -> Shift Arithmetic/1

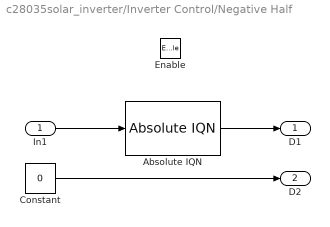
== system c28035solar_inverter/Inverter Control/Negative Half ==
  In1 : Inport
  Enable : EnablePort
  Absolute IQN : tiiqmathlib/Absolute IQN
      settings: SourceProductBaseCode=TIC2000
  Constant : Constant  Value=0  OutDataTypeStr=fixdt(1,32,24)
  D1 : Outport  VectorParamsAs1DForOutWhenUnconnected=off
  D2 : Outport  Port=2  VectorParamsAs1DForOutWhenUnconnected=off
  wires:
  In1/1 -> Absolute IQN/1
  Constant/1 -> D2/1
  Absolute IQN/1 -> D1/1

== system c28035solar_inverter/Inverter Control/Positive Half ==
  In1 : Inport
  Enable : EnablePort
  Constant : Constant  Value=0  OutDataTypeStr=fixdt(1,32,24)
  D1 : Outport  VectorParamsAs1DForOutWhenUnconnected=off
  D2 : Outport  Port=2  VectorParamsAs1DForOutWhenUnconnected=off
  wires:
  Constant/1 -> D1/1
  In1/1 -> D2/1

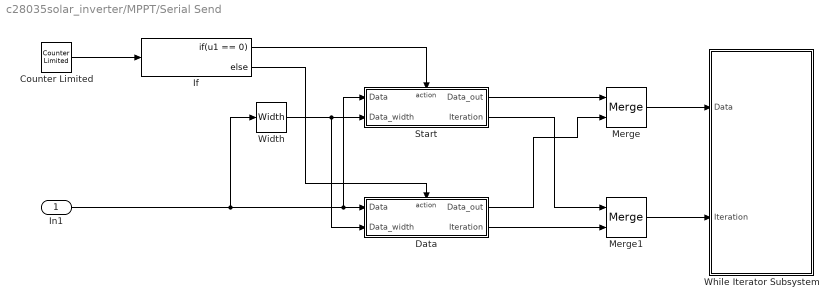
== system c28035solar_inverter/MPPT/Serial Send ==
  In1 : Inport
  Counter Limited : simulink/Sources/Counter Limited  uplimit=9  tsamp=-1
  Data : Subsystem  TreatAsAtomicUnit=on
  If : If  IfExpression=u1 == 0
  Merge : Merge
  Merge1 : Merge
  Start : Subsystem  TreatAsAtomicUnit=on
  While Iterator Subsystem : Subsystem  TreatAsAtomicUnit=on
  Width : Width  OutDataTypeMode=All ports same datatype  DataType=uint16
  wires:
  In1/1 -> Data/1(Data), Start/1(Data), Width/1
  Width/1 -> Start/2(Data_width), Data/2(Data_width)
  Data/2(Iteration) -> Merge1/2
  Start/2(Iteration) -> Merge1/1
  Merge1/1 -> While Iterator Subsystem/2(Iteration)
  Merge/1 -> While Iterator Subsystem/1(Data)
  Data/1(Data_out) -> Merge/2
  Start/1(Data_out) -> Merge/1
  Counter Limited/1 -> If/1
  If/2 -> Data/Action
  If/1 -> Start/Action

== system c28035solar_inverter/DC-DC Boost Controller/PI_Controller_Optimized/Integrator ==
  u : Inport
  Sum : Sum  Inputs=|++  RndMeth=Simplest  OutDataTypeStr=Inherit: Same as first input
  Unit Delay : UnitDelay  SampleTime=-1  HasFrameUpgradeWarning=on
      settings: AttributesFormatString=State = %<StateName>\nInitialValue = %<InitialCondition>
  y : Outport  VectorParamsAs1DForOutWhenUnconnected=off
  wires:
  u/1 -> Sum/1
  Unit Delay/1 -> Sum/2
  Sum/1 -> y/1, Unit Delay/1

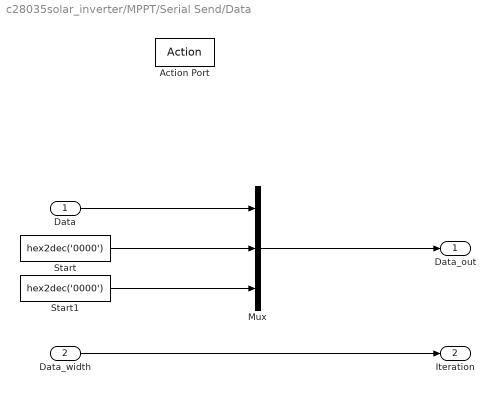
== system c28035solar_inverter/MPPT/Serial Send/Data ==
  Data : Inport
  Data_width : Inport  Port=2
  Action Port : ActionPort  ActionPortLabel=else
  Mux : Mux  Inputs=3
  Start : Constant  Value=hex2dec('0000')  OutDataTypeStr=uint16
  Start1 : Constant  Value=hex2dec('0000')  OutDataTypeStr=uint16
  Data_out : Outport  VectorParamsAs1DForOutWhenUnconnected=off
  Iteration : Outport  Port=2  VectorParamsAs1DForOutWhenUnconnected=off
  wires:
  Start1/1 -> Mux/3
  Data_width/1 -> Iteration/1
  Data/1 -> Mux/1
  Mux/1 -> Data_out/1
  Start/1 -> Mux/2

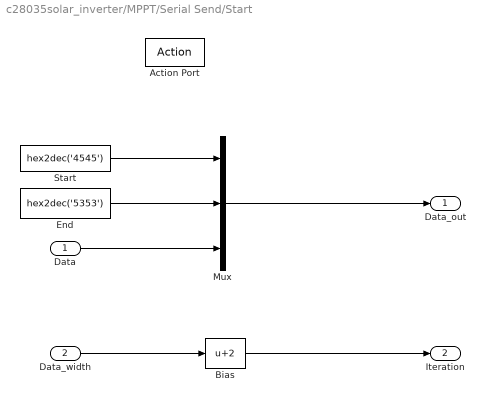
== system c28035solar_inverter/MPPT/Serial Send/Start ==
  Data : Inport
  Data_width : Inport  Port=2
  Action Port : ActionPort  ActionPortLabel=if(u1 == 0)
  Bias : Bias  Bias=2
  End : Constant  Value=hex2dec('5353')  OutDataTypeStr=uint16
  Mux : Mux  Inputs=3
  Start : Constant  Value=hex2dec('4545')  OutDataTypeStr=uint16
  Data_out : Outport  VectorParamsAs1DForOutWhenUnconnected=off
  Iteration : Outport  Port=2  VectorParamsAs1DForOutWhenUnconnected=off
  wires:
  Start/1 -> Mux/1
  Data/1 -> Mux/3
  Bias/1 -> Iteration/1
  Data_width/1 -> Bias/1
  Mux/1 -> Data_out/1
  End/1 -> Mux/2

== system c28035solar_inverter/MPPT/Serial Send/While Iterator Subsystem ==
  Data : Inport
  Iteration : Inport  Port=2
  Add : Sum  Inputs=+-  OutDataTypeStr=Inherit: Same as first input
  Index Vector : MultiPortSwitch  Inputs=1
  SCI Transmit : c280xlib/SCI Transmit  sciModule=A  dataHead=''  dataTail=''  postInterrupt=off  numFifo=1
  While Iterator : WhileIterator  MaxIters=-1  WhileBlockType=do-while  ShowIterationPort=on  OutputDataType=int16
  wires:
  While Iterator/1 -> Add/2, Index Vector/1
  Data/1 -> Index Vector/2
  Index Vector/1 -> SCI Transmit/1
  Add/1 -> While Iterator/1
  Iteration/1 -> Add/1

== stateflow chart c28035solar_inverter/MPPT/P&O MPPT ==
  state DisableMPPT
    during:
    Vref = VrefCmd;
    Vref_prev = VrefCmd;
  state EnableMPPT
    state Compute_Power
      entry:
      P = V*I;
    state Calculate_Difference
      entry:
      deltaP = P - Pprev;
      deltaV = V - Vprev;
    state Decrement_Vref
      entry:
      Vref = Vref_prev - delV;
    state Increment_Vref
      entry:
      Vref = Vref_prev + delV;
    state Save_PreviousValues
      entry:
      Pprev = P; Vprev = V;
    state Clamp_VrefMax
      entry:
      Vref = VrefMax;
    state Clamp_VrefMin
      entry:
      Vref = VrefMin;
    (default) -> Compute_Power : {Vref_prev = 0.8*V;}
    (junction 96) -> Compute_Power
    (junction 106) -> (junction 96) : {Vref_prev = Vref;}
    Compute_Power -> Calculate_Difference
    Calculate_Difference -> (junction 103) [order 1] : [deltaP < 0]
    Calculate_Difference -> (junction 104) [order 2] : [deltaP >= 0]
    (junction 103) -> Increment_Vref [order 2] : [deltaV < 0]
    (junction 104) -> Decrement_Vref [order 1] : [deltaV <= 0]
    (junction 103) -> Decrement_Vref [order 1] : [deltaV >= 0]
    (junction 104) -> Increment_Vref [order 2] : [deltaV > 0]
    Decrement_Vref -> Save_PreviousValues
    Increment_Vref -> Save_PreviousValues
    Save_PreviousValues -> (junction 106) [order 3]
    (junction 73) -> (junction 106)
    Save_PreviousValues -> Clamp_VrefMax [order 1] : [Vref >= VrefMax]
    Save_PreviousValues -> Clamp_VrefMin [order 2] : [Vref <= VrefMin]
    Clamp_VrefMax -> (junction 88)
    Clamp_VrefMin -> (junction 98)
    (junction 88) -> (junction 98)
    (junction 98) -> (junction 73)
  (default) -> DisableMPPT
  (junction 89) -> DisableMPPT
  EnableMPPT -> (junction 89) : [MPPT ~= 1]
  DisableMPPT -> EnableMPPT : [MPPT == 1 && V >= 4]
  data: P local single =single(0); deltaP local single =single(0); Pprev local single =single(0); Vprev local single =single(0); deltaV local single =single(0); V input; I input; Vref output single; Vref_prev local; VrefCmd input; MPPT input; delV input single; VrefMax constant single =single(28); VrefMin constant single =single(1)
